simulink subsystem "F550_calcFaultInjectedPWM"  (R2024a)
settings: Solver=VariableStepAuto  StartTime=0.0  StopTime=10.0  RelTol=1e-3
settings Model: Creator=CNU_UASG  LastModifiedBy=CNU_UASG

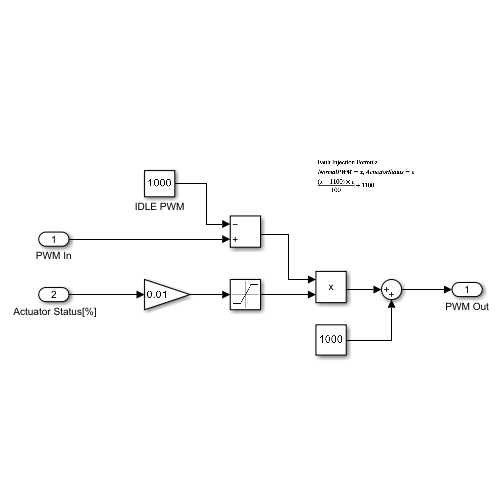
[thumbnail: Simulink's stored preview of the top-level diagram]
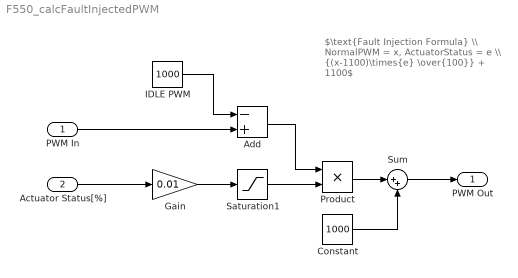
== system F550_calcFaultInjectedPWM ==
  note: $\text{Fault Injection Formula} \\ NormalPWM = x, ActuatorStatus = e \\ {(x-1100)\times{e} \over{100}} + 1100$
  PWM In : Inport
  " Actuator Status[%]" : Inport  Port=2
  Add : Sum  Inputs=-+
  Constant : Constant  Value=1000
  Gain : Gain  Gain=0.01
  IDLE PWM : Constant  Value=1000
  Product : Product
  Saturation1 : Saturate  UpperLimit=1  LowerLimit=0
  Sum : Sum  Inputs=|++
  PWM Out : Outport
  wires:
  Add/1 -> Product/1
  Gain/1 -> Saturation1/1
  " Actuator Status[%]"/1 -> Gain/1
  Product/1 -> Sum/1
  Constant/1 -> Sum/2
  PWM In/1 -> Add/2
  Saturation1/1 -> Product/2
  IDLE PWM/1 -> Add/1
  Sum/1 -> PWM Out/1
